simulink model "bh_wheel_dynamics_COMPARE_hand_SEME_to_simscape"  (R2020b)
settings: Solver=ode45  StartTime=0.0  StopTime=80  FixedStep=0.001  RelTol=1e-6  EnableMultiTasking=on
undefined symbols (not defined in the file or in its folder): d, Ic_xx_val, m, r, sigbuilder_block, X, Y, Z
libraries: simulink_extras x12, sm_lib x11, nesl_utility x3
settings Model: Creator=bhorton  LastModifiedBy=bhorton
settings SolverCC: ZeroCrossAlgorithm=Adaptive
settings DataIOCC: SaveOutput=off  SignalLogging=off  DSMLogging=off  VisualizeSimOutput=off  SaveTime=off  ReturnWorkspaceOutputs=off
settings OptimizationCC: LifeSpan=inf
settings DebuggingCC: AllowSymbolicDim=off  SFUnexpectedBacktrackingDiag=warning  SFNoUnconditionalDefaultTransitionDiag=warning  SFExecutionAtInitializationDiag=none  ArithmeticOperatorsInVariantConditions=warning
settings ModelReferenceCC: PropagateSignalLabelsOutOfModel=off
settings SFSimCC: SimUseLocalCustomCode=off  CustomCodeUndefinedFunction=UseInterfaceOnly
settings RTWCC: RTWUseLocalCustomCode=off
settings CodeAppCC: StateflowObjectComments=on
settings GRTTargetCC: TargetLangStandard=C89/C90 (ANSI)
settings ConfigComp: CovMetricSettings=dw  CovSaveCumulativeToWorkspaceVar=on  CovSaveSingleToWorkspaceVar=on  CovExternalEMLEnable=off
settings SimscapeCC: SimscapeNormalizeSystem=off
settings ExplorerConfigSet: InternalSimMechanicsExplorerSettings="<ExplorerConfiguration><canonicalview>default</canonicalview><AnimationSetting><BasePlaybackSpeed>1.0</BasePlaybackSpeed><PlaybackSpeedFactor>1.0</PlaybackSpeedFactor></AnimationSetting><TilePanel><TileInfo><Tiles Columns=\"2\" Count=\"4\" Rows=\"2\"><Column Weight=\"0.5\"/><Column Weight=\"0.5\"/><Row Weight=\"0.4994\"/><Row Weight=\"0.5006\"/><Tile Height=\"1\" Width=\"1\" X=\"0\" Y=\"0\"/><Tile Height=\"1\" Width=\"1\" X=\"0\" Y=\"1\"/><Tile Height=\"1\" Width=\"1\" X=\"1\" Y=\"0\"/><Tile Height=\"1\" Width=\"1\" X=\"1\" Y=\"1\"/></Tiles></TileInfo><SceneInfo><SceneViewer><BGColor><R>0.60000002384185791</R><G>0.60000002384185791</G><B>0.60000002384185791</B></BGColor><Camera><DoPerspective>off</DoPerspective><Position><X>-0.0548914633691310883</X><Y>-1.00972235202789307</Y><Z>-0.000268854200839330204</Z></Position><Center><X>-0.0548914633691310883</X><Y>-0.00972235202789306641</Y><Z>-0.000268854200839330204</Z></Center><Up><X>0</X><Y>-0</Y><Z>1</Z></Up><ViewLimDist>1</ViewLimDist><YLim>0.242988618314266214</YLim><XLim>0.415537839409340637</XLim></Camera></SceneViewer><SceneViewer><BGColor><R>0.60000002384185791</R><G>0.60000002384185791</G><B>0.60000002384185791</B></BGColor><Camera><DoPerspective>off</DoPerspective><Position><X>-0.0668795574456453323</X><Y>-0.0157359018921852112</Y><Z>0.999887213110924433</Z></Position><Center><X>-0.0668795574456453323</X><Y>-0.0157359018921852112</Y><Z>-0.000112786889075566776</Z></Center><Up><X>0</X><Y>1</Y><Z>-0</Z></Up><ViewLimDist>1</ViewLimDist><YLim>0.265369449853897099</YLim><XLim>0.452794061297793038</XLim></Camera></SceneViewer><SceneViewer><BGColor><R>0.60000002384185791</R><G>0.60000002384185791</G><B>0.60000002384185791</B></BGColor><Camera><DoPerspective>off</DoPerspective><Position><X>0.933120416477322578</X><Y>-0.0157359018921852112</Y><Z>-0.000112786889075566776</Z></Position><Center><X>-0.0668795835226774216</X><Y>-0.0157359018921852112</Y><Z>-0.000112786889075566776</Z></Center><Up><X>-0</X><Y>0</Y><Z>1</Z></Up><ViewLimDist>1</ViewLimDist><YLim>0.269939221739768975</YLim><XLim>0.461626399424638623</XLim></Camera></SceneViewer><SceneViewer><BGColor><R>0.60000002384185791</R><G>0.60000002384185791</G><B>0.60000002384185791</B></BGColor><Camera><DoPerspective>off</DoPerspective><Position><X>0.509141991470968391</X><Y>-0.593086175670118343</Y><Z>0.577237479619849725</Z></Position><Center><X>-0.0682082777186574229</X><Y>-0.0157359064804924592</Y><Z>-0.000112789569776162307</Z></Center><Up><X>-0.408248290463863073</X><Y>0.408248290463863073</Y><Z>0.816496580927726145</Z></Up><ViewLimDist>1</ViewLimDist><YLim>0.277322931885719326</YLim><XLim>0.473190025033704942</XLim></Camera></SceneViewer></SceneInfo></TilePanel><MechEditorPanel><Cameras/><GfxPanelCameraMap/><VideoCreator><PlaybackSpeedRatio>1.0</PlaybackSpeedRatio><FrameRate>30</FrameRate><VideoFormat>Motion JPEG AVI</VideoFormat><FrameSize>auto</FrameSize></VideoCreator></MechEditorPanel></ExplorerConfiguration>"

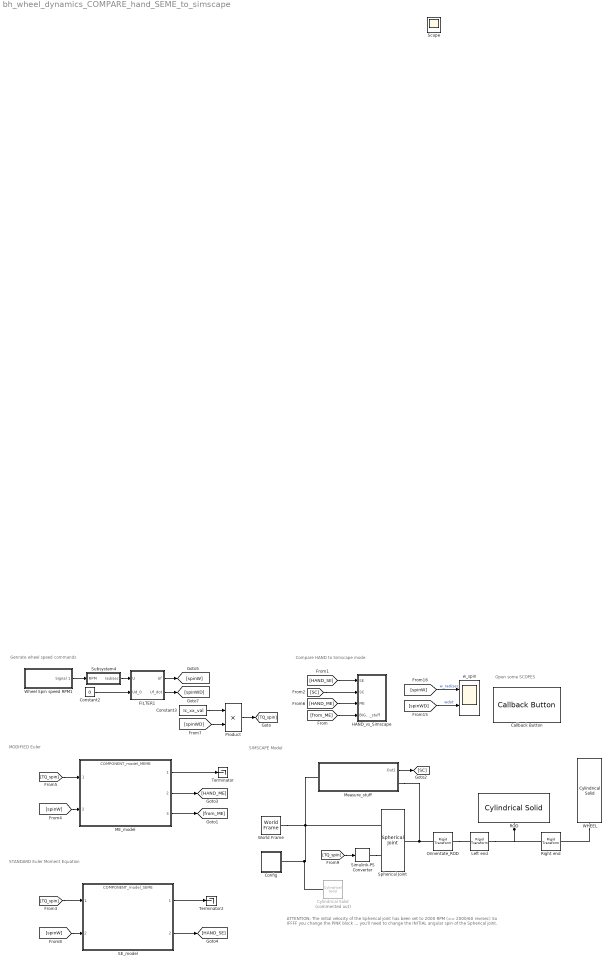
== system bh_wheel_dynamics_COMPARE_hand_SEME_to_simscape ==
  note: Open some SCOPES
  note: ATTENTION:
      | The initial velocity of the Spherical joint has been set to 2000 RPM (== 2000/60 rev/sec)
      | So IFFFF you change the PINK block ... you'll need to change the INITIAL angular spin
      | of the Spherical joint.
  note: SIMSCAPE Model
  note: Compare HAND to Simscape mode
  note: Genrate wheel speed commands
  note: STANDARD Euler Moment Equation
  note: MODIFIED Euler
  Callback Button : CallbackButton  ButtonText=Open the SCOPES
      settings: ClickFcn=|
      | my_scope = [bdroot,'/HAND_vs_Simscape/HAND_SE vs Simscape'];
      | open_system(my_scope)
      | 
      | 
      | my_scope = [bdroot,'/w_spin'];
      | open_system(my_scope)
  Config : Subsystem
  Constant2 : Constant  Value=0
  Constant3 : Constant  Value=Ic_xx_val
  Cylindrical Solid : sm_lib/Body Elements/Cylindrical Solid  Commented=on  GraphicAmbientColor=[0.15 0.15 0.15 1.0]  BasedOnType=Density  CenterOfMass=[0 0 0]  CenterOfMassUnits=m  GraphicDiffuseColor=[0.0 1.0 0.2]  CylinderLength=1  CylinderLengthUnits=m  CylinderRadius=0.02  CylinderRadiusUnits=m  Density=1000  DensityUnits=kg/m^3  DoExposeReferenceFrame=on  GraphicEmissiveColor=[0.0 0.0 0.0 1.0]  ExportEntireGeometry=off  SerializedFrames=<Frames><Frame><Id>Frame1</Id><Value><Name>TOP</Name><Origin><Source>GeometricFeature</Source><FeatureName>top surface</FeatureName></Origin><PrimaryAxis><DefinedDirection>+Z</DefinedDirection><Source>ReferenceFrame</Source><SourceDirection>+Z</SourceDirection><FeatureName></FeatureName></PrimaryAxis><SecondaryAxis><DefinedDirection>+X</DefinedDirection><Source>ReferenceFrame</Source><SourceDirection>+X</SourceDirection><FeatureName></FeatureName></SecondaryAxis></Value></Frame></Frames>  MarkerShape=Sphere  MarkerSize=10  GraphicType=FromGeometry  InertiaType=CalculateFromGeometry  Mass=1  MassUnits=kg  MomentsOfInertia=[1 1 1]  MomentsOfInertiaUnits=kg*m^2  GraphicOpacity=1.0  ProductsOfInertia=[0 0 0]  ProductsOfInertiaUnits=kg*m^2  GraphicShininess=75  GraphicSpecularColor=[0.5 0.5 0.5 1.0]  GraphicVisPropType=SimpleVisualProperties
  FILTER1 : Subsystem
  HAND_vs_Simscape : Subsystem
  Left end : sm_lib/Frames and Transforms/Rigid Transform  TranslationMethod=StandardAxis  TranslationStandardOffset=d/2  TranslationLengthUnit=m  TranslationStandardAxis=+Z  TranslationCartesianOffset=[0 0 0]  TranslationROffset=0  TranslationROffsetUnits=m  TranslationZOffset=0  TranslationZOffsetUnits=m  TranslationThetaOffset=0  TranslationThetaOffsetUnits=deg  RotationMethod=None  RotationAngleUnits=deg  RotationStandardAxis=+Z  RotationAngle=0.0  RotationArbitraryAxis=[0 0 1]  FollAlignAxisA=+X  BaseAlignAxisA=+Y  FollAlignAxisB=+Y  BaseAlignAxisB=+Z  RotationSequenceAxes=FollowerAxes  RotationSequence=XYX  RotationSequenceAngles=[0 0 0]  RotationSequenceAnglesUnits=deg  RotationMatrix=[1 0 0; 0 1 0; 0 0 1]
  ME_model : ModelReference  ModelNameDialog=COMPONENT_model_MEME.slx  SimulationMode=Normal  ModelReferenceVersion=2.1
  Measure_stuff : Subsystem
  Orinentate_ROD : sm_lib/Frames and Transforms/Rigid Transform  TranslationMethod=None  TranslationStandardOffset=0  TranslationLengthUnit=m  TranslationStandardAxis=+Z  TranslationCartesianOffset=[0 0 0]  TranslationROffset=0  TranslationROffsetUnits=m  TranslationZOffset=0  TranslationZOffsetUnits=m  TranslationThetaOffset=0  TranslationThetaOffsetUnits=deg  RotationMethod=AlignedAxes  RotationAngleUnits=deg  RotationStandardAxis=+Z  RotationAngle=0.0  RotationArbitraryAxis=[0 0 1]  FollAlignAxisA=+Z  BaseAlignAxisA=+X  FollAlignAxisB=+X  BaseAlignAxisB=-Z  RotationSequenceAxes=FollowerAxes  RotationSequence=XYX  RotationSequenceAngles=[0 0 0]  RotationSequenceAnglesUnits=deg  RotationMatrix=[1 0 0; 0 1 0; 0 0 1]
  Product : Product
  ROD : sm_lib/Body Elements/Cylindrical Solid  GraphicAmbientColor=[0.15 0.15 0.15 1.0]  BasedOnType=Mass  CenterOfMass=[0 0 0]  CenterOfMassUnits=m  GraphicDiffuseColor=[1.0 0.6 0.6]  CylinderLength=d  CylinderLengthUnits=m  CylinderRadius=0.01  CylinderRadiusUnits=m  Density=1000  DensityUnits=kg/(m^3)  DoExposeReferenceFrame=on  GraphicEmissiveColor=[0.0 0.0 0.0 1.0]  ExportEntireGeometry=off  SerializedFrames=<Frames/>  MarkerShape=Sphere  MarkerSize=10  GraphicType=FromGeometry  InertiaType=CalculateFromGeometry  Mass=1e-6  MassUnits=kg  MomentsOfInertia=[1 1 1]  MomentsOfInertiaUnits=kg*m^2  GraphicOpacity=1.0  ProductsOfInertia=[0 0 0]  ProductsOfInertiaUnits=kg*m^2  GraphicShininess=75  GraphicSpecularColor=[0.5 0.5 0.5 1.0]  GraphicVisPropType=SimpleVisualProperties
  Right end : sm_lib/Frames and Transforms/Rigid Transform  TranslationMethod=StandardAxis  TranslationStandardOffset=d/2  TranslationLengthUnit=m  TranslationStandardAxis=+Z  TranslationCartesianOffset=[0 0 0]  TranslationROffset=0  TranslationROffsetUnits=m  TranslationZOffset=0  TranslationZOffsetUnits=m  TranslationThetaOffset=0  TranslationThetaOffsetUnits=deg  RotationMethod=None  RotationAngleUnits=deg  RotationStandardAxis=+Z  RotationAngle=0.0  RotationArbitraryAxis=[0 0 1]  FollAlignAxisA=+X  BaseAlignAxisA=+Y  FollAlignAxisB=+Y  BaseAlignAxisB=+Z  RotationSequenceAxes=FollowerAxes  RotationSequence=XYX  RotationSequenceAngles=[0 0 0]  RotationSequenceAnglesUnits=deg  RotationMatrix=[1 0 0; 0 1 0; 0 0 1]
  SE_model : ModelReference  ModelNameDialog=COMPONENT_model_SEME.slx  SimulationMode=Normal  ModelReferenceVersion=1.562
  Simulink-PS Converter : nesl_utility/Simulink-PS Converter  PhysicalDomain=network_engine_domain  SubClassName=ps_input  LeftPortType=input  RightPortType=output  PseudoPeriodic=off  Frequencies=[]  NoiseDistribution=none  NoiseParameters=[]  Unit=N*m  AffineConversion=off  FilteringAndDerivatives=provide  SimscapeFilterOrder=1  InputFilterTimeConstant=0.001  UdotUserProvided=0
  Spherical Joint : sm_lib/Joints/Spherical Joint  JointMode=Normal  SenseConstraintForce=off  SenseConstraintForceX=off  SenseConstraintForceY=off  SenseConstraintForceZ=off  SenseConstraintTorque=off  SenseConstraintTorqueX=off  SenseConstraintTorqueY=off  SenseConstraintTorqueZ=off  SenseTotalForce=off  SenseTotalForceX=off  SenseTotalForceY=off  SenseTotalForceZ=off  SenseTotalTorque=off  SenseTotalTorqueX=off  SenseTotalTorqueY=off  SenseTotalTorqueZ=off  CompositeWrenchDir=FollowerOnBase  CompositeWrenchFrame=BaseFrame  DefPosRotationMethod=None  DefPosRotationAngleUnits=deg  DefPosRotationStandardAxis=+Z  DefPosRotationAngle=0.0  DefPosRotationArbitraryAxis=[0 0 1]  DefPosFollAlignAxisA=+X  DefPosBaseAlignAxisA=+Y  DefPosFollAlignAxisB=+Y  DefPosBaseAlignAxisB=+Z  DefPosRotationSequenceAxes=FollowerAxes  DefPosRotationSequence=XYX  DefPosRotationSequenceAngles=[0 0 0]  DefPosRotationSequenceAnglesUnits=deg  DefPosRotationMatrix=[1 0 0; 0 1 0; 0 0 1]  EqPosRotationMethod=None  EqPosRotationAngleUnits=deg  EqPosRotationStandardAxis=+Z  EqPosRotationAngle=0.0  EqPosRotationArbitraryAxis=[0 0 1]  EqPosFollAlignAxisA=+X  EqPosBaseAlignAxisA=+Y  EqPosFollAlignAxisB=+Y  EqPosBaseAlignAxisB=+Z  EqPosRotationSequenceAxes=FollowerAxes  EqPosRotationSequence=XYX  EqPosRotationSequenceAngles=[0 0 0]  EqPosRotationSequenceAnglesUnits=deg  EqPosRotationMatrix=[1 0 0; 0 1 0; 0 0 1]  SpringStiffness=0  SpringStiffnessUnits=N*m/deg  DampingCoefficient=0  DampingCoefficientUnits=N*m/(deg/s)  ActuateTorqueX=on  ActuateTorqueY=off  ActuateTorqueZ=off  ActuateTorque=off  TorqueActuationMode=InputTorque  MotionActuationMode=ComputedMotion  ActuationFrame=FollowerFrame  SensePosition=off  SenseVelocityX=off  SenseVelocityY=off  SenseVelocityZ=off  SenseVelocity=off  SenseAccelerationX=off  SenseAccelerationY=off  SenseAccelerationZ=off  SenseAcceleration=off  SenseTorqueX=off  SenseTorqueY=off  SenseTorqueZ=off  SenseTorqueForce=off  SenseLowerLimitTorqueMag=off  SenseUpperLimitTorqueMag=off  SensingFrame=BaseFrame  LowerLimitSpecify=off  LowerLimitBound=15  LowerLimitBoundUnits=deg  LowerLimitStiffness=1e4  LowerLimitStiffnessUnits=N*m/deg  LowerLimitDamping=10  LowerLimitDampingUnits=N*m/(deg/s)  LowerLimitTransitionRegionWidth=0.1  LowerLimitTransitionRegionWidthUnits=deg  UpperLimitSpecify=off  UpperLimitBound=45  UpperLimitBoundUnits=deg  UpperLimitStiffness=1e4  UpperLimitStiffnessUnits=N*m/deg  UpperLimitDamping=10  UpperLimitDampingUnits=N*m/(deg/s)  UpperLimitTransitionRegionWidth=0.1  UpperLimitTransitionRegionWidthUnits=deg  PositionTargetRotationMethod=None  PositionTargetRotationAngleUnits=deg  PositionTargetRotationStandardAxis=+Z  PositionTargetRotationAngle=0.0  PositionTargetRotationArbitraryAxis=[0 0 1]  PositionTargetFollAlignAxisA=+X  PositionTargetBaseAlignAxisA=+Y  PositionTargetFollAlignAxisB=+Y  PositionTargetBaseAlignAxisB=+Z  PositionTargetRotationSequenceAxes=FollowerAxes  PositionTargetRotationSequence=XYX  PositionTargetRotationSequenceAngles=[0 0 0]  PositionTargetRotationSequenceAnglesUnits=deg  PositionTargetRotationMatrix=[1 0 0; 0 1 0; 0 0 1]  PositionTargetSpecify=off  PositionTargetPriority=High  VelocityTargetValue=[(2000/60) 0 0]  VelocityTargetValueUnits=rev/s  VelocityTargetSpecify=on  VelocityTargetPriority=High  VelocityTargetInFollowerFrame=on
      settings: AttributesFormatString=|
      | Init_VEL = %<VelocityTargetValue>
      |  (%<VelocityTargetValueUnits>)
  Subsystem4 : Subsystem
  Terminator : Terminator
  Terminator2 : Terminator
  WHEEL : sm_lib/Body Elements/Cylindrical Solid  GraphicAmbientColor=[0.15 0.15 0.15 1.0]  BasedOnType=Mass  CenterOfMass=[0 0 0]  CenterOfMassUnits=m  GraphicDiffuseColor=[0.6 0.6 1.0]  CylinderLength=t  CylinderLengthUnits=m  CylinderRadius=r  CylinderRadiusUnits=m  Density=m/(t * pi*r^2)  DensityUnits=kg/(m^3)  DoExposeReferenceFrame=on  GraphicEmissiveColor=[0.0 0.0 0.0 1.0]  ExportEntireGeometry=off  SerializedFrames=<Frames/>  MarkerShape=Sphere  MarkerSize=10  GraphicType=FromGeometry  InertiaType=CalculateFromGeometry  Mass=m  MassUnits=kg  MomentsOfInertia=[1 1 1]  MomentsOfInertiaUnits=kg*m^2  GraphicOpacity=1.0  ProductsOfInertia=[0 0 0]  ProductsOfInertiaUnits=kg*m^2  GraphicShininess=75  GraphicSpecularColor=[0.5 0.5 0.5 1.0]  GraphicVisPropType=SimpleVisualProperties
  Wheel Spin speed RPM1 : Subsystem  Tag=STV Subsys  LoadFcn=sigbuilder_block('load');  StartFcn=sigbuilder_block('start');  StopFcn=sigbuilder_block('stop');  ClipboardFcn=sigbuilder_block('clipboard');  mask(Sigbuilder block){tuvar=[0:10]}
      mask help: Simulink:masks:SigbuilderBlock_MD
      mask init:
      | if ~strcmp(get_param(bdroot(gcbh),'SimulationStatus'),'stopped') tuvar = sigbuilder_block('maskInit'); end
      settings: CopyFcn=sigbuilder_block('copy');  DeleteFcn=sigbuilder_block('delete');  ModelCloseFcn=sigbuilder_block('modelClose');  PreSaveFcn=sigbuilder_block('preSave');  PauseFcn=sigbuilder_block('pause');  ContinueFcn=sigbuilder_block('continue');  NameChangeFcn=sigbuilder_block('namechange');  OpenFcn=sigbuilder_block('open',[6 6 1428 740.25 ]);  CloseFcn=sigbuilder_block('close');
      mask Display: plot(0, 0, 100, 100,[2, 2, 32, 32, 2], [68, 8, 8, 68, 68],[32, 2], [38, 38], [32, 19, 2],[53, 60, 44], [32, 17, 17, 2],[16, 16, 31, 31]);txt = getActiveGroup(gcbh);text(2, 100, txt,'verticalAlignment', 'top');
  World Frame : sm_lib/Frames and Transforms/World Frame
  w_spin : Scope  NumInputPorts=2
  Scope : Scope
  wires:
  [HAND_SE] -> HAND_vs_Simscape/1(SE)
  [SC] -> HAND_vs_Simscape/2(SC)
  [TQ_spin] -> Simulink-PS Converter/1
  [HAND_ME] -> HAND_vs_Simscape/3(ME)
  [TQ_spin] -> SE_model/1
  Product/1 -> [TQ_spin]
  [spinW] -> w_spin/1  "w_rad/sec"
  [spinWD] -> w_spin/2  "wdot"
  Subsystem4/1(rad/sec) -> FILTER1/1(U)
  Constant3/1 -> Product/1
  Wheel Spin speed RPM1/1(Signal 1) -> Subsystem4/1(RPM)
  [spinW] -> ME_model/2
  [spinWD] -> Product/2
  FILTER1/2(Uf_dot) -> [spinWD]
  SE_model/1 -> Terminator2/1
  Constant2/1 -> FILTER1/2(Ud_0)
  SE_model/2 -> [HAND_SE]
  ME_model/1 -> Terminator/1
  [spinW] -> SE_model/2
  ME_model/2 -> [HAND_ME]
  FILTER1/1(Uf) -> [spinW]
  [TQ_spin] -> ME_model/1
  ME_model/3 -> [from_ME]
  [from_ME] -> HAND_vs_Simscape/4(BIG_Omega_stuff)
  Measure_stuff/1(Out1) -> [SC]
  connections:
  Orinentate_ROD/LConn1 -- Measure_stuff/RConn1 -- Spherical Joint/RConn1
  World Frame/RConn1 -- Measure_stuff/LConn1 -- Cylindrical Solid/LConn1 -- Config/LConn1 -- Spherical Joint/LConn1
  ROD/RConn1 -- Right end/LConn1 -- Left end/RConn1
  Simulink-PS Converter/RConn1 -- Spherical Joint/LConn2
  Orinentate_ROD/RConn1 -- Left end/LConn1
  WHEEL/RConn1 -- Right end/RConn1

== system bh_wheel_dynamics_COMPARE_hand_SEME_to_simscape/Config ==
  Mechanism Configuration : sm_lib/Utilities/Mechanism Configuration  UniformGravity=Constant  GravityVector=[0 0 -9.81]  GravityVectorUnits=m/s^2  GravityUnits=m/s^2  LinearizationDelta=0.001  JointModeTransitionNonlinearIterations=2
  Solver Configuration : nesl_utility/Solver Configuration  PhysicalDomain=network_engine_domain  SubClassName=solver  LeftPortType=input  RightPortType=generic  Tones=[]  Harmonics=[]  SimulateNoise=off  Profile=off  UseLocalSampling=off  EnableSwitchedLinearOptims=on  FrequencyDomain=off  UseCCode=off  RelTol=0.001  AbsTol=1e-06  MinStep=1e-09  ToWorkspace=off  RevertToSquareIcSolve=off  NumHomotopyIterations=100  PhasorMode=off  PhasorModeNumHarmonics=1  DoDC=off  ResidualTolerance=1e-09  UseLocalSolver=off  LocalSolverChoice=NE_BACKWARD_EULER_ADVANCER  LocalSolverSampleTime=0.001  DoFixedCost=off  MaxNonlinIter=3  MaxModeIter=2  ComputeImpulses=off  ImpulseIterations=2  LinearAlgebra=Sparse  EquationFormulation=NE_TIME_EF  DelaysMemoryBudget=1024  AutomaticFiltering=on  FilteringTimeConstant=0.001  PartitionStorageMethod=AS_NEEDED  PartitionMemoryBudget=1024  PartitionMethod=FAST
  W : PMIOPort  Side=Left
  connections:
  Solver Configuration/RConn1 -- W/RConn1 -- Mechanism Configuration/RConn1

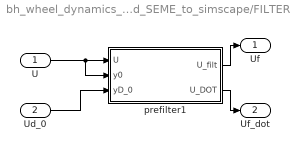
== system bh_wheel_dynamics_COMPARE_hand_SEME_to_simscape/FILTER1 ==
  U : Inport
  Ud_0 : Inport  Port=2
  prefilter1 : Subsystem  mask(Derivative Estimation){wn=2*pi*5, p=1}
      mask prompts: wn "Natural frequency, wn (rad/sec)"; p "Damping ratio, p"
      mask help:
      | A simple derivative estimator using a 2nd order representation between input and output.
      |
      | The integrators use a discrete FORWARd Euler rule, and a sample time needs to be specified.
      mask init:
      | str1 = sprintf('wn = %.2f', wn);
      | str2 = sprintf('p  = %.2f', p);
      | %str3 = sprintf('dt = %.2f', dt);
      | %str = char(str1,str2,str3);
      | %str3 = sprintf('dt = %.2f', dt);
      | str = char(str1,str2);
      mask Display: disp(str)
  Uf : Outport  VectorParamsAs1DForOutWhenUnconnected=off
  Uf_dot : Outport  Port=2  VectorParamsAs1DForOutWhenUnconnected=off
  wires:
  Ud_0/1 -> prefilter1/3(yD_0)
  prefilter1/2(U_DOT) -> Uf_dot/1
  prefilter1/1(U_filt) -> Uf/1
  U/1 -> prefilter1/2(y0), prefilter1/1(U)

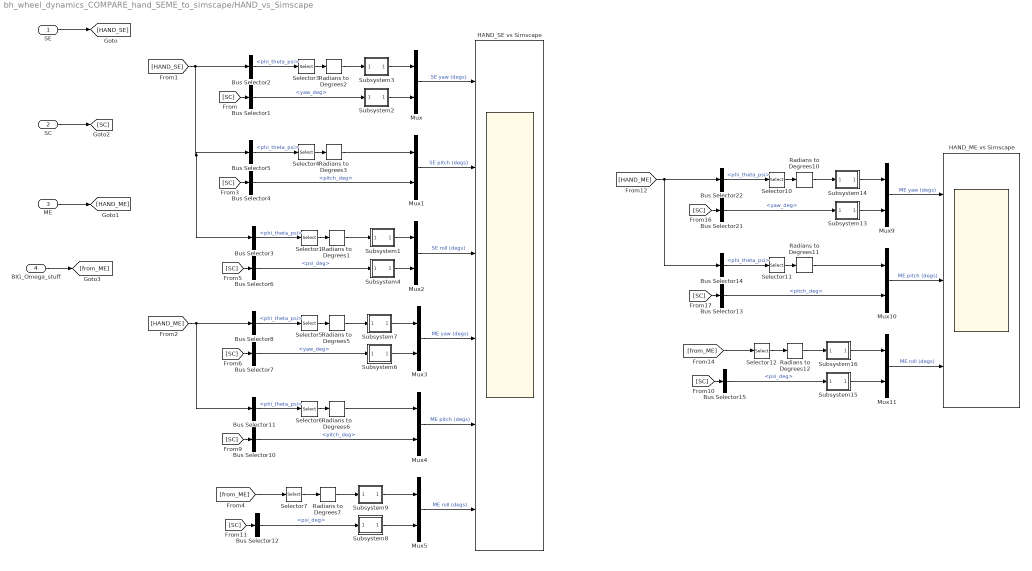
== system bh_wheel_dynamics_COMPARE_hand_SEME_to_simscape/HAND_vs_Simscape ==
  SE : Inport
  SC : Inport  Port=2
  ME : Inport  Port=3
  BIG_Omega_stuff : Inport  Port=4
  Bus Selector1 : BusSelector  OutputSignals=yaw_deg
  Bus Selector10 : BusSelector  OutputSignals=pitch_deg
  Bus Selector{2..3,5,8,11,14,22} (7 alike) : BusSelector  OutputSignals=phi_theta_psi
  Bus Selector12 : BusSelector  OutputSignals=psi_deg
  Bus Selector13 : BusSelector  OutputSignals=pitch_deg
  Bus Selector15 : BusSelector  OutputSignals=psi_deg
  Bus Selector21 : BusSelector  OutputSignals=yaw_deg
  Bus Selector4 : BusSelector  OutputSignals=pitch_deg
  Bus Selector6 : BusSelector  OutputSignals=psi_deg
  Bus Selector7 : BusSelector  OutputSignals=yaw_deg
  HAND_ME vs Simscape : Scope  NumInputPorts=3
  HAND_SE vs Simscape : Scope  NumInputPorts=6
  Mux{,1..5,9..11} (9 alike) : Mux  Inputs=2
  Radians to Degrees{1..3,5..7,10..12} (9 alike) : simulink_extras/Transformations/Radians to Degrees
  Selector1 : Selector  InputPortWidth=3  IndexOptions=Index vector (dialog)  Indices=3  OutputSizes=1
  Selector10 : Selector  InputPortWidth=3  IndexOptions=Index vector (dialog)  Indices=1  OutputSizes=1
  Selector11 : Selector  InputPortWidth=3  IndexOptions=Index vector (dialog)  Indices=2  OutputSizes=1
  Selector12 : Selector  InputPortWidth=2  IndexOptions=Index vector (dialog)  Indices=2  OutputSizes=1
  Selector3 : Selector  InputPortWidth=3  IndexOptions=Index vector (dialog)  Indices=1  OutputSizes=1
  Selector4 : Selector  InputPortWidth=3  IndexOptions=Index vector (dialog)  Indices=2  OutputSizes=1
  Selector5 : Selector  InputPortWidth=3  IndexOptions=Index vector (dialog)  Indices=1  OutputSizes=1
  Selector6 : Selector  InputPortWidth=3  IndexOptions=Index vector (dialog)  Indices=2  OutputSizes=1
  Selector7 : Selector  InputPortWidth=2  IndexOptions=Index vector (dialog)  Indices=2  OutputSizes=1
  Subsystem1 : Subsystem
      mask Display: disp(sprintf('Mod\n360'))
  Subsystem13 : Subsystem
      mask Display: disp(sprintf('Mod\n360'))
  Subsystem14 : Subsystem
      mask Display: disp(sprintf('Mod\n360'))
  Subsystem15 : Subsystem
      mask Display: disp(sprintf('Mod\n360'))
  Subsystem16 : Subsystem
      mask Display: disp(sprintf('Mod\n360'))
  Subsystem2 : Subsystem
      mask Display: disp(sprintf('Mod\n360'))
  Subsystem3 : Subsystem
      mask Display: disp(sprintf('Mod\n360'))
  Subsystem4 : Subsystem
      mask Display: disp(sprintf('Mod\n360'))
  Subsystem6 : Subsystem
      mask Display: disp(sprintf('Mod\n360'))
  Subsystem7 : Subsystem
      mask Display: disp(sprintf('Mod\n360'))
  Subsystem8 : Subsystem
      mask Display: disp(sprintf('Mod\n360'))
  Subsystem9 : Subsystem
      mask Display: disp(sprintf('Mod\n360'))
  wires:
  SE/1 -> [HAND_SE]
  SC/1 -> [SC]
  [SC] -> Bus Selector1/1
  Bus Selector1/1 -> Subsystem2/1(In1)  "<yaw_deg>"
  Bus Selector2/1 -> Selector3/1  "<phi_theta_psi>"
  Selector3/1 -> Radians to Degrees2/1
  Radians to Degrees2/1 -> Subsystem3/1(In1)
  Subsystem2/1(Out1) -> Mux/2
  Subsystem3/1(Out1) -> Mux/1
  Radians to Degrees3/1 -> Mux1/1
  Bus Selector4/1 -> Mux1/2  "<pitch_deg>"
  Bus Selector5/1 -> Selector4/1  "<phi_theta_psi>"
  Selector4/1 -> Radians to Degrees3/1
  [SC] -> Bus Selector4/1
  Mux1/1 -> HAND_SE vs Simscape/2  "SE pitch (degs)"
  Mux/1 -> HAND_SE vs Simscape/1  "SE yaw (degs)"
  Mux2/1 -> HAND_SE vs Simscape/3  "SE roll (degs)"
  Radians to Degrees1/1 -> Subsystem1/1(In1)
  Selector1/1 -> Radians to Degrees1/1
  [HAND_SE] -> Bus Selector3/1, Bus Selector5/1, Bus Selector2/1
  Bus Selector3/1 -> Selector1/1  "<phi_theta_psi>"
  [SC] -> Bus Selector6/1
  Bus Selector6/1 -> Subsystem4/1(In1)  "<psi_deg>"
  Subsystem1/1(Out1) -> Mux2/1
  Subsystem4/1(Out1) -> Mux2/2
  ME/1 -> [HAND_ME]
  Subsystem9/1(Out1) -> Mux5/1
  [HAND_ME] -> Bus Selector11/1, Bus Selector8/1
  Subsystem8/1(Out1) -> Mux5/2
  Bus Selector12/1 -> Subsystem8/1(In1)  "<psi_deg>"
  Mux3/1 -> HAND_SE vs Simscape/4  "ME yaw (degs)"
  [SC] -> Bus Selector12/1
  Selector6/1 -> Radians to Degrees6/1
  Mux4/1 -> HAND_SE vs Simscape/5  "ME pitch (degs)"
  [SC] -> Bus Selector10/1
  Radians to Degrees5/1 -> Subsystem7/1(In1)
  Mux5/1 -> HAND_SE vs Simscape/6  "ME roll (degs)"
  Bus Selector11/1 -> Selector6/1  "<phi_theta_psi>"
  [SC] -> Bus Selector7/1
  Bus Selector8/1 -> Selector5/1  "<phi_theta_psi>"
  Selector5/1 -> Radians to Degrees5/1
  Subsystem6/1(Out1) -> Mux3/2
  Radians to Degrees6/1 -> Mux4/1
  Bus Selector10/1 -> Mux4/2  "<pitch_deg>"
  Bus Selector7/1 -> Subsystem6/1(In1)  "<yaw_deg>"
  Subsystem7/1(Out1) -> Mux3/1
  BIG_Omega_stuff/1 -> [from_ME]
  Radians to Degrees7/1 -> Subsystem9/1(In1)
  [from_ME] -> Selector7/1
  Selector7/1 -> Radians to Degrees7/1
  Selector12/1 -> Radians to Degrees12/1
  Radians to Degrees12/1 -> Subsystem16/1(In1)
  [from_ME] -> Selector12/1
  Mux10/1 -> HAND_ME vs Simscape/2  "ME pitch (degs)"
  Mux11/1 -> HAND_ME vs Simscape/3  "ME roll (degs)"
  Selector10/1 -> Radians to Degrees10/1
  Bus Selector21/1 -> Subsystem13/1(In1)  "<yaw_deg>"
  Subsystem13/1(Out1) -> Mux9/2
  Bus Selector22/1 -> Selector10/1  "<phi_theta_psi>"
  Subsystem14/1(Out1) -> Mux9/1
  [HAND_ME] -> Bus Selector14/1, Bus Selector22/1
  Bus Selector13/1 -> Mux10/2  "<pitch_deg>"
  [SC] -> Bus Selector21/1
  [SC] -> Bus Selector15/1
  Bus Selector15/1 -> Subsystem15/1(In1)  "<psi_deg>"
  Subsystem15/1(Out1) -> Mux11/2
  [SC] -> Bus Selector13/1
  Mux9/1 -> HAND_ME vs Simscape/1  "ME yaw (degs)"
  Radians to Degrees10/1 -> Subsystem14/1(In1)
  Bus Selector14/1 -> Selector11/1  "<phi_theta_psi>"
  Radians to Degrees11/1 -> Mux10/1
  Selector11/1 -> Radians to Degrees11/1
  Subsystem16/1(Out1) -> Mux11/1

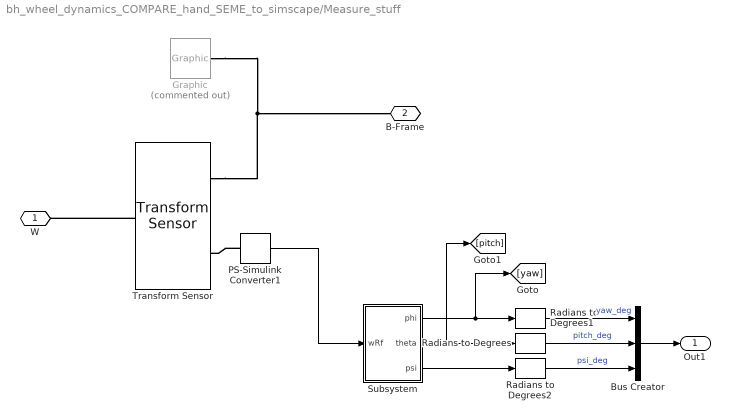
== system bh_wheel_dynamics_COMPARE_hand_SEME_to_simscape/Measure_stuff ==
  Bus Creator : BusCreator  Inputs=3
  Graphic : sm_lib/Body Elements/Graphic  Commented=on  GraphicType=Marker  MarkerShape=Frame  MarkerSize=45  GraphicVisPropType=SimpleVisualProperties  GraphicDiffuseColor=[0.0 0.0 0.0]  GraphicSpecularColor=[0.5 0.5 0.5 1.0]  GraphicAmbientColor=[0.15 0.15 0.15 1.0]  GraphicEmissiveColor=[0.0 0.0 0.0 1.0]  GraphicShininess=75  GraphicOpacity=1.0
  PS-Simulink Converter1 : nesl_utility/PS-Simulink Converter  PhysicalDomain=network_engine_domain  SubClassName=ps_output  LeftPortType=input  RightPortType=output  PseudoPeriodic=off  Frequencies=[]  Unit=1  AffineConversion=off
  Radians to Degrees : simulink_extras/Transformations/Radians to Degrees
  Radians to Degrees1 : simulink_extras/Transformations/Radians to Degrees
  Radians to Degrees2 : simulink_extras/Transformations/Radians to Degrees
  Subsystem : Subsystem
  Transform Sensor : sm_lib/Frames and Transforms/Transform Sensor  MeasurementFrame=World  SenseAngle=off  SenseAxis=off  SenseAngle1=off  SenseAngle2=off  SenseAngle3=off  SenseQ=off  SenseR=on  SenseOmegaX=off  SenseOmegaY=off  SenseOmegaZ=off  SenseOmega1=off  SenseOmega2=off  SenseOmega3=off  SenseQDot=off  SenseRDot=off  SenseAlphaX=off  SenseAlphaY=off  SenseAlphaZ=off  SenseAlpha1=off  SenseAlpha2=off  SenseAlpha3=off  SenseQDDot=off  SenseRDDot=off  SenseX=off  SenseY=off  SenseZ=off  SenseRad=off  SenseAzim=off  SenseDist=off  SenseInc=off  SenseXDot=off  SenseYDot=off  SenseZDot=off  SenseRadDot=off  SenseAzimDot=off  SenseDistDot=off  SenseIncDot=off  SenseXDDot=off  SenseYDDot=off  SenseZDDot=off  SenseRadDDot=off  SenseAzimDDot=off  SenseDistDDot=off  SenseIncDDot=off
  W : PMIOPort  Side=Left
  B-Frame : PMIOPort  Port=2  Side=Right
  Out1 : Outport
  wires:
  Radians to Degrees/1 -> Bus Creator/2  "pitch_deg"
  Radians to Degrees1/1 -> Bus Creator/1  "yaw_deg"
  Subsystem/3(psi) -> Radians to Degrees2/1
  Radians to Degrees2/1 -> Bus Creator/3  "psi_deg"
  PS-Simulink Converter1/1 -> Subsystem/1(wRf)
  Subsystem/1(phi) -> [yaw], Radians to Degrees1/1
  Subsystem/2(theta) -> [pitch], Radians to Degrees/1
  Bus Creator/1 -> Out1/1
  connections:
  Transform Sensor/LConn1 -- W/RConn1
  Transform Sensor/RConn1 -- Graphic/RConn1 -- B-Frame/RConn1
  PS-Simulink Converter1/LConn1 -- Transform Sensor/RConn2

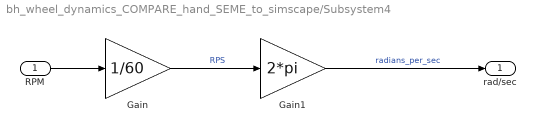
== system bh_wheel_dynamics_COMPARE_hand_SEME_to_simscape/Subsystem4 ==
  RPM : Inport
  Gain : Gain  Gain=1/60
  Gain1 : Gain  Gain=2*pi
  rad/sec : Outport  VectorParamsAs1DForOutWhenUnconnected=off
  wires:
  RPM/1 -> Gain/1
  Gain/1 -> Gain1/1  "RPS"
  Gain1/1 -> rad/sec/1  "radians_per_sec"

== system bh_wheel_dynamics_COMPARE_hand_SEME_to_simscape/Wheel Spin speed RPM1 ==
  Demux : Demux  Tag=STV Demux  Outputs=1
      settings: DisplayOption=none
  FromWs : FromWorkspace  Tag=STV FromWs  VariableName=tuvar
      SigBuilderData=|
      | common.afterFinalStr = 'Extrapolate'
      | common.sampleTime = 0
      | dataSet(1).timeRange = [0 60]
      | dataSet(1).name = 'RAMP_DOWN'
      | dataSet(2).timeRange = [0 80]
      | dataSet(2).name = 'STAIRCASE_DOWN'
      | dataSet(3).timeRange = [0 60]
      | dataSet(3).name = 'STAIRCASE_UP'
      | sbobj.Groups(1).Name = 'RAMP_DOWN'
      | sbobj.Groups(1).Signals.Name = 'Signal 1'
      | sbobj.Groups(1).Signals.XData = [0 60]
      | sbobj.Groups(1).Signals.YData = [2000 0]
      | sbobj.Groups(1).TimeRange = [0 60]
      | sbobj.Groups(2).Name = 'STAIRCASE_DOWN'
      | sbobj.Groups(2).Signals.Name = 'Signal 1'
      | sbobj.Groups(2).Signals.XData = [0 10.1 10.1 20 20 30 30 39.9 39.9 49.9 49.9 60.2 60.2 70 70 80]
      | sbobj.Groups(2).Signals.YData = [2000 2000 1500 1500 1000 1000 750 750 500 500 150 150 60 60 0 0]
      | sbobj.Groups(2).TimeRange = [0 80]
      | sbobj.Groups(3).Name = 'STAIRCASE_UP'
      | sbobj.Groups(3).Signals.Name = 'Signal 1'
      | sbobj.Groups(3).Signals.XData = [0 9.9 9.9 19.9 19.9 30.1 30.1 39.9 39.9 49.9 49.9 60]
      | sbobj.Groups(3).Signals.YData = [2000 2000 2200 2200 2400 2400 2610 2610 1800 1800 1600 1600]
      | sbobj.Groups(3).TimeRange = [0 60]
  Signal 1 : Outport  Tag=STV Outport  VectorParamsAs1DForOutWhenUnconnected=off
  wires:
  Demux/1 -> Signal 1/1
  FromWs/1 -> Demux/1

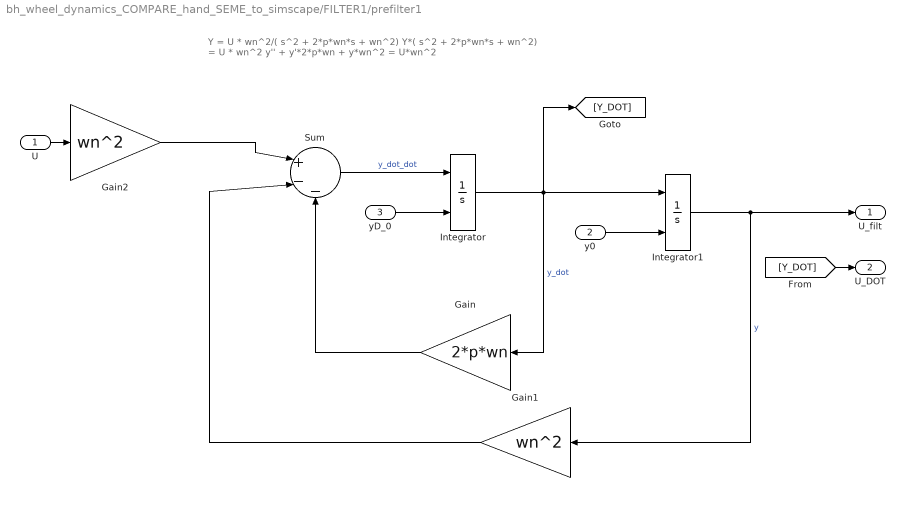
== system bh_wheel_dynamics_COMPARE_hand_SEME_to_simscape/FILTER1/prefilter1 ==
  note: Y = U *     wn^2/( s^2 + 2*p*wn*s + wn^2)
      | Y*( s^2 + 2*p*wn*s + wn^2) = U * wn^2
      |
      | y'' + y'*2*p*wn + y*wn^2 = U*wn^2
  U : Inport
  y0 : Inport  Port=2
  yD_0 : Inport  Port=3
  Gain : Gain  Gain=2*p*wn
  Gain1 : Gain  Gain=wn^2
  Gain2 : Gain  Gain=wn^2
  Integrator : Integrator  InitialConditionSource=external
  Integrator1 : Integrator  InitialConditionSource=external
  Sum : Sum  Inputs=|+--
  U_filt : Outport  VectorParamsAs1DForOutWhenUnconnected=off
  U_DOT : Outport  Port=2  VectorParamsAs1DForOutWhenUnconnected=off
  wires:
  Integrator/1 -> [Y_DOT], Gain/1, Integrator1/1  "y_dot"
  Sum/1 -> Integrator/1  "y_dot_dot"
  Integrator1/1 -> Gain1/1, U_filt/1  "y"
  U/1 -> Gain2/1
  Gain2/1 -> Sum/1
  Gain/1 -> Sum/3
  Gain1/1 -> Sum/2
  [Y_DOT] -> U_DOT/1
  yD_0/1 -> Integrator/2
  y0/1 -> Integrator1/2

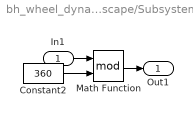
== system bh_wheel_dynamics_COMPARE_hand_SEME_to_simscape/HAND_vs_Simscape/Subsystem1 ==
  In1 : Inport
  Constant2 : Constant  Value=360
  Math Function : Math  Operator=mod  SignedPower=on  SaturateOnIntegerOverflow=on
  Out1 : Outport  VectorParamsAs1DForOutWhenUnconnected=off
  wires:
  Math Function/1 -> Out1/1
  In1/1 -> Math Function/1
  Constant2/1 -> Math Function/2

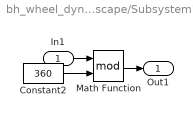
== system bh_wheel_dynamics_COMPARE_hand_SEME_to_simscape/HAND_vs_Simscape/Subsystem13 ==
  In1 : Inport
  Constant2 : Constant  Value=360
  Math Function : Math  Operator=mod  SignedPower=on  SaturateOnIntegerOverflow=on
  Out1 : Outport  VectorParamsAs1DForOutWhenUnconnected=off
  wires:
  Math Function/1 -> Out1/1
  In1/1 -> Math Function/1
  Constant2/1 -> Math Function/2

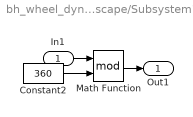
== system bh_wheel_dynamics_COMPARE_hand_SEME_to_simscape/HAND_vs_Simscape/Subsystem14 ==
  In1 : Inport
  Constant2 : Constant  Value=360
  Math Function : Math  Operator=mod  SignedPower=on  SaturateOnIntegerOverflow=on
  Out1 : Outport  VectorParamsAs1DForOutWhenUnconnected=off
  wires:
  Math Function/1 -> Out1/1
  In1/1 -> Math Function/1
  Constant2/1 -> Math Function/2

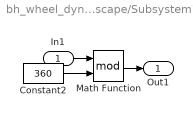
== system bh_wheel_dynamics_COMPARE_hand_SEME_to_simscape/HAND_vs_Simscape/Subsystem15 ==
  In1 : Inport
  Constant2 : Constant  Value=360
  Math Function : Math  Operator=mod  SignedPower=on  SaturateOnIntegerOverflow=on
  Out1 : Outport  VectorParamsAs1DForOutWhenUnconnected=off
  wires:
  Math Function/1 -> Out1/1
  In1/1 -> Math Function/1
  Constant2/1 -> Math Function/2

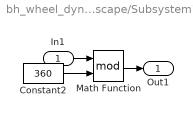
== system bh_wheel_dynamics_COMPARE_hand_SEME_to_simscape/HAND_vs_Simscape/Subsystem16 ==
  In1 : Inport
  Constant2 : Constant  Value=360
  Math Function : Math  Operator=mod  SignedPower=on  SaturateOnIntegerOverflow=on
  Out1 : Outport  VectorParamsAs1DForOutWhenUnconnected=off
  wires:
  Math Function/1 -> Out1/1
  In1/1 -> Math Function/1
  Constant2/1 -> Math Function/2

== system bh_wheel_dynamics_COMPARE_hand_SEME_to_simscape/HAND_vs_Simscape/Subsystem2 ==
  In1 : Inport
  Constant2 : Constant  Value=360
  Math Function : Math  Operator=mod  SignedPower=on  SaturateOnIntegerOverflow=on
  Out1 : Outport  VectorParamsAs1DForOutWhenUnconnected=off
  wires:
  Math Function/1 -> Out1/1
  In1/1 -> Math Function/1
  Constant2/1 -> Math Function/2

== system bh_wheel_dynamics_COMPARE_hand_SEME_to_simscape/HAND_vs_Simscape/Subsystem3 ==
  In1 : Inport
  Constant2 : Constant  Value=360
  Math Function : Math  Operator=mod  SignedPower=on  SaturateOnIntegerOverflow=on
  Out1 : Outport  VectorParamsAs1DForOutWhenUnconnected=off
  wires:
  Math Function/1 -> Out1/1
  In1/1 -> Math Function/1
  Constant2/1 -> Math Function/2

== system bh_wheel_dynamics_COMPARE_hand_SEME_to_simscape/HAND_vs_Simscape/Subsystem4 ==
  In1 : Inport
  Constant2 : Constant  Value=360
  Math Function : Math  Operator=mod  SignedPower=on  SaturateOnIntegerOverflow=on
  Out1 : Outport  VectorParamsAs1DForOutWhenUnconnected=off
  wires:
  Math Function/1 -> Out1/1
  In1/1 -> Math Function/1
  Constant2/1 -> Math Function/2

== system bh_wheel_dynamics_COMPARE_hand_SEME_to_simscape/HAND_vs_Simscape/Subsystem6 ==
  In1 : Inport
  Constant2 : Constant  Value=360
  Math Function : Math  Operator=mod  SignedPower=on  SaturateOnIntegerOverflow=on
  Out1 : Outport  VectorParamsAs1DForOutWhenUnconnected=off
  wires:
  Math Function/1 -> Out1/1
  In1/1 -> Math Function/1
  Constant2/1 -> Math Function/2

== system bh_wheel_dynamics_COMPARE_hand_SEME_to_simscape/HAND_vs_Simscape/Subsystem7 ==
  In1 : Inport
  Constant2 : Constant  Value=360
  Math Function : Math  Operator=mod  SignedPower=on  SaturateOnIntegerOverflow=on
  Out1 : Outport  VectorParamsAs1DForOutWhenUnconnected=off
  wires:
  Math Function/1 -> Out1/1
  In1/1 -> Math Function/1
  Constant2/1 -> Math Function/2

== system bh_wheel_dynamics_COMPARE_hand_SEME_to_simscape/HAND_vs_Simscape/Subsystem8 ==
  In1 : Inport
  Constant2 : Constant  Value=360
  Math Function : Math  Operator=mod  SignedPower=on  SaturateOnIntegerOverflow=on
  Out1 : Outport  VectorParamsAs1DForOutWhenUnconnected=off
  wires:
  Math Function/1 -> Out1/1
  In1/1 -> Math Function/1
  Constant2/1 -> Math Function/2

== system bh_wheel_dynamics_COMPARE_hand_SEME_to_simscape/HAND_vs_Simscape/Subsystem9 ==
  In1 : Inport
  Constant2 : Constant  Value=360
  Math Function : Math  Operator=mod  SignedPower=on  SaturateOnIntegerOverflow=on
  Out1 : Outport  VectorParamsAs1DForOutWhenUnconnected=off
  wires:
  Math Function/1 -> Out1/1
  In1/1 -> Math Function/1
  Constant2/1 -> Math Function/2

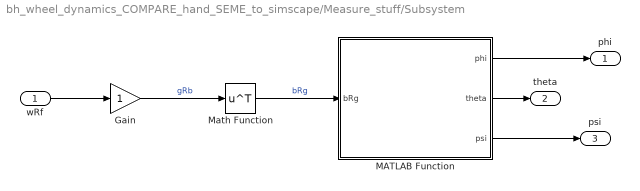
== system bh_wheel_dynamics_COMPARE_hand_SEME_to_simscape/Measure_stuff/Subsystem ==
  wRf : Inport
  Gain : Gain
  MATLAB Function : MATLAB Function  TreatAsAtomicUnit=on
  Math Function : Math  Operator=transpose  SignedPower=on  SaturateOnIntegerOverflow=on
  phi : Outport  VectorParamsAs1DForOutWhenUnconnected=off
  theta : Outport  Port=2  VectorParamsAs1DForOutWhenUnconnected=off
  psi : Outport  Port=3  VectorParamsAs1DForOutWhenUnconnected=off
  wires:
  wRf/1 -> Gain/1
  Gain/1 -> Math Function/1  "gRb"
  Math Function/1 -> MATLAB Function/1(bRg)  "bRg"
  MATLAB Function/1(phi) -> phi/1
  MATLAB Function/2(theta) -> theta/1
  MATLAB Function/3(psi) -> psi/1

== matlab function bh_wheel_dynamics_COMPARE_hand_SEME_to_simscape/Measure_stuff/Subsystem/MATLAB Function ==
  data: bRg input; phi output; theta output; psi output
function [phi, theta, psi] = calc_bRg(bRg)
%#codegen

% bRg = [ ...
%                               cos(phi)*cos(theta),                              cos(theta)*sin(phi),         -sin(theta);
%  cos(phi)*sin(psi)*sin(theta) - cos(psi)*sin(phi), cos(phi)*cos(psi) + sin(phi)*sin(psi)*sin(theta), cos(theta)*sin(psi);
%  sin(phi)*sin(psi) + cos(phi)*cos(psi)*sin(theta), cos(psi)*sin(phi)*sin(theta) - cos(phi)*sin(psi), cos(psi)*cos(theta);
%  ];

phi   = 0; 
theta = 0;
psi   = 0;

theta = -asin(  bRg(1,3) ); % so +/- pi/2 range

phi   = atan2( bRg(1,2) , bRg(1,1)  );  % so +/- pi range
psi   = atan2( bRg(2,3) , bRg(3,3)  );  % so +/- pi range


% THE_TAN_PHI =  bRg(1,2) / bRg(1,1);
% 
% phi   = atan2( THE_TAN_PHI  );  % so +/- pi range
% 
% THE_TAN_PSI =  bRg(2,3) / bRg(3,3);
% 
% psi   = atan2( THE_TAN_PSI  );  % so +/- pi range


% convert to [0 2pi]
if(phi < 0)   
    phi = pi + (pi - abs(phi) );   
end

if(psi < 0)   
    psi = pi + (pi - abs(psi) );   
end

end %function
